simulink model "c28x_i2c_eeprom"  (R2021b)
settings: Solver=FixedStepDiscrete  StartTime=0.0  StopTime=inf  RelTol=1e-3  EnableMultiTasking=on
libraries: simulink x3, c280xlib x3, demo_controls x1, idelinklib_common x1
settings Model: SimulationMode=external  ExtModeTrigDuration=8  Creator=The MathWorks, Inc.  LastModifiedBy=The MathWorks, Inc.
settings SolverCC: AlgebraicLoopSolver=TrustRegion
settings DataIOCC: ReturnWorkspaceOutputs=off
settings OptimizationCC: DefaultUnderspecifiedDataType=single  PassReuseOutputArgsAs=Individual arguments  MaxStackSize=512  EfficientTunableParamExpr=on
settings DebuggingCC: ParameterTunabilityLossMsg=error  SFMachineParentedDataDiag=warning  ArithmeticOperatorsInVariantConditions=warning
settings HardwareCC: ProdBitPerChar=16  ProdBitPerInt=16  ProdBitPerPointer=32  ProdBitPerSizeT=32  ProdBitPerPtrDiffT=32  ProdLargestAtomicInteger=Integer  ProdLargestAtomicFloat=None  ProdWordSize=16  ProdLongLongMode=on  ProdHWDeviceType=Texas Instruments->C2000
settings SFSimCC: SimUseLocalCustomCode=off  CustomCodeUndefinedFunction=UseInterfaceOnly
settings RTWCC: Description=Embedded Coder  SystemTargetFile=ert.tlc  HardwareBoard=TI Delfino F2833x  TemplateMakefile=ert_default_tmf  GenerateReport=on  RTWUseLocalCustomCode=off  Toolchain=Texas Instruments Code Composer Studio (C2000)  IncludeHyperlinkInReport=on  LaunchReport=on  GenerateTraceInfo=on  GenerateTraceReport=on  GenerateTraceReportSl=on  GenerateTraceReportSf=on  GenerateTraceReportEml=on
settings CodeAppCC: ForceParamTrailComments=on  IgnoreCustomStorageClasses=off  OperatorAnnotations=on  SimulinkDataObjDesc=on  SFDataObjDesc=on  MATLABFcnDesc=on  InsertBlockDesc=on  StateflowObjectComments=on  MATLABSourceComments=on
settings ERTTargetCC: CodeReplacementLibrary=TI C28x  ExtModeTransport=4  ExtModeStaticAlloc=on  ExtModeStaticAllocSize=5000  ExtModeMexFile=ext_xcp  ExtModeIntrfLevel=Level2 - Open

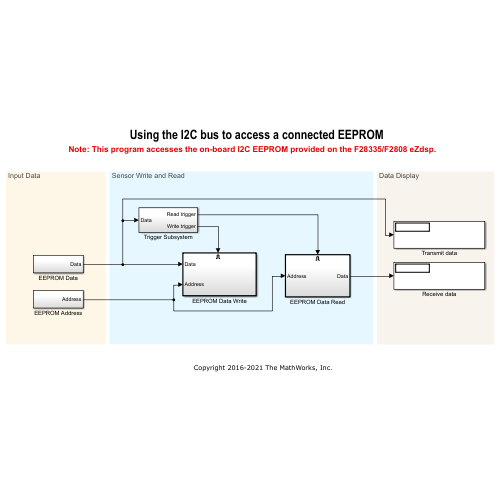
[thumbnail: Simulink's stored preview of the top-level diagram]
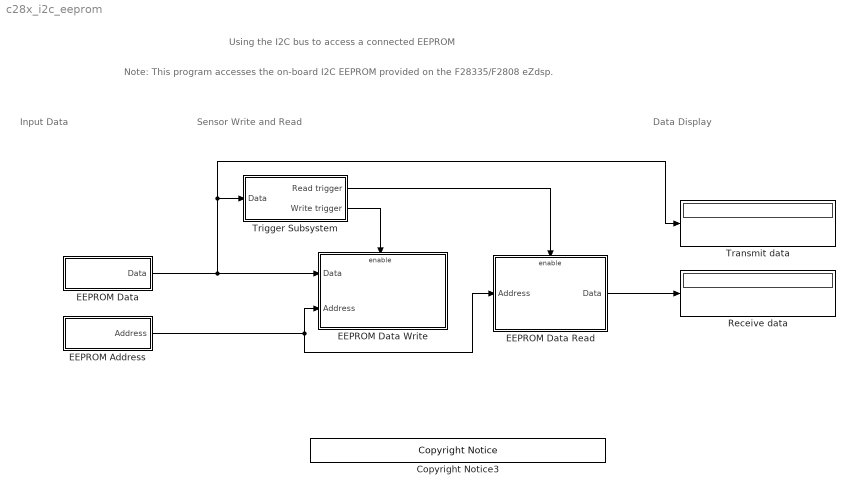
== system c28x_i2c_eeprom ==
  note: Note: This program accesses the on-board I2C EEPROM provided on the F28335/F2808 eZdsp.
  note: Using the I2C bus to access a connected EEPROM
  note: Data Display
  note: Sensor Write and Read
  note: Input Data
  Copyright Notice3 : demo_controls/Copyright Notice  year=2016  prod=tic2000
      settings: SourceProductBaseCode=ME
  EEPROM Address : Subsystem
  EEPROM Data : Subsystem
  EEPROM Data Read : Subsystem
  EEPROM Data Write : Subsystem  TreatAsAtomicUnit=on
  Receive data : Display
  Transmit data : Display
  Trigger Subsystem : Subsystem
  wires:
  EEPROM Data Read/1(Data) -> Receive data/1
  EEPROM Address/1(Address) -> EEPROM Data Read/1(Address), EEPROM Data Write/2(Address)
  EEPROM Data/1(Data) -> Transmit data/1, Trigger Subsystem/1(Data), EEPROM Data Write/1(Data)
  Trigger Subsystem/1(Read trigger) -> EEPROM Data Read/Enable
  Trigger Subsystem/2(Write trigger) -> EEPROM Data Write/Enable

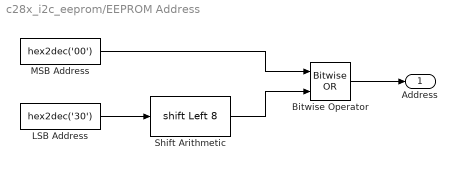
== system c28x_i2c_eeprom/EEPROM Address ==
  Bitwise Operator : simulink/Logic and Bit Operations/Bitwise Operator  logicop=OR  UseBitMask=off  NumInputPorts=2  BitMask=bin2dec('11011001')  BitMaskRealWorld=Stored Integer
  LSB Address : Constant  Value=hex2dec('30')  OutDataTypeStr=uint16  SampleTime=-1
  MSB Address : Constant  Value=hex2dec('00')  OutDataTypeStr=uint16  SampleTime=-1
  Shift Arithmetic : ArithShift  BitShiftNumber=8  BitShiftDirection=Left
  Address : Outport  VectorParamsAs1DForOutWhenUnconnected=off
  wires:
  LSB Address/1 -> Shift Arithmetic/1
  MSB Address/1 -> Bitwise Operator/1
  Shift Arithmetic/1 -> Bitwise Operator/2
  Bitwise Operator/1 -> Address/1

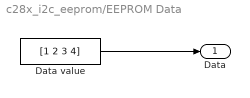
== system c28x_i2c_eeprom/EEPROM Data ==
  Data value : Constant  Value=[1 2 3 4]  OutDataTypeStr=uint16  SampleTime=-1
  Data : Outport  VectorParamsAs1DForOutWhenUnconnected=off
  wires:
  Data value/1 -> Data/1

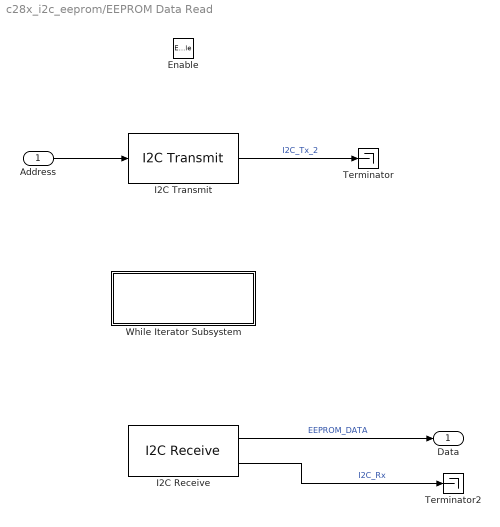
== system c28x_i2c_eeprom/EEPROM Data Read ==
  Address : Inport
  Enable : EnablePort
  I2C Receive : c280xlib/I2C Receive  Priority=3  selectModule=I2C_A  addrFormat=7-Bit addressing  saSource=Specify via dialog  SAR=hex2dec('50')  bitCount=8  dataLength=4  initValue=0  NACK=off  STP=on  STR=on  sampleTime=0.2  dataType=uint16
      settings: SourceProductBaseCode=TIC2000
  I2C Transmit : c280xlib/I2C Transmit  Priority=1  selectModule=I2C_A  addrFormat=7-Bit addressing  saSource=Specify via dialog  SAR=hex2dec('50')  bitCount=8  STP=off  RM=off  STR=on
      settings: SourceProductBaseCode=TIC2000
  Terminator : Terminator
  Terminator2 : Terminator
  While Iterator Subsystem : Subsystem  Priority=2  TreatAsAtomicUnit=on
  Data : Outport  VectorParamsAs1DForOutWhenUnconnected=off
  wires:
  I2C Receive/2 -> Terminator2/1  "I2C_Rx"
  I2C Transmit/1 -> Terminator/1  "I2C_Tx_2"
  Address/1 -> I2C Transmit/1
  I2C Receive/1 -> Data/1  "EEPROM_DATA"

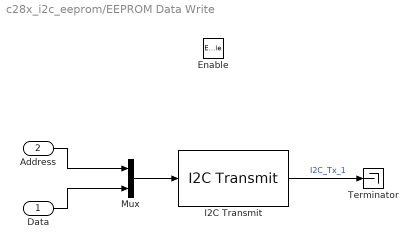
== system c28x_i2c_eeprom/EEPROM Data Write ==
  Data : Inport
  Address : Inport  Port=2
  Enable : EnablePort
  I2C Transmit : c280xlib/I2C Transmit  Priority=1  selectModule=I2C_A  addrFormat=7-Bit addressing  saSource=Specify via dialog  SAR=hex2dec('50')  bitCount=8  STP=on  RM=off  STR=on
      settings: SourceProductBaseCode=TIC2000
  Mux : Mux  Inputs=2
  Terminator : Terminator
  wires:
  I2C Transmit/1 -> Terminator/1  "I2C_Tx_1"
  Mux/1 -> I2C Transmit/1
  Data/1 -> Mux/2
  Address/1 -> Mux/1

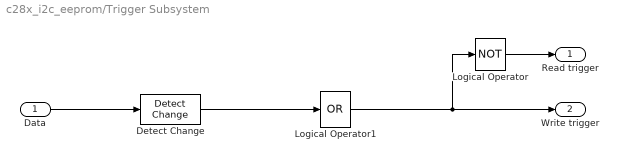
== system c28x_i2c_eeprom/Trigger Subsystem ==
  Data : Inport
  Detect Change : simulink/Logic and Bit Operations/Detect Change  vinit=0  OutDataTypeStr=boolean
  Logical Operator : Logic  Operator=NOT  AllPortsSameDT=off  OutDataTypeStr=boolean
  Logical Operator1 : Logic  Operator=OR  Inputs=1  AllPortsSameDT=off  OutDataTypeStr=boolean
  Read trigger : Outport  VectorParamsAs1DForOutWhenUnconnected=off
  Write trigger : Outport  Port=2  VectorParamsAs1DForOutWhenUnconnected=off
  wires:
  Data/1 -> Detect Change/1
  Detect Change/1 -> Logical Operator1/1
  Logical Operator1/1 -> Logical Operator/1, Write trigger/1
  Logical Operator/1 -> Read trigger/1

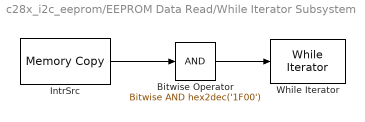
== system c28x_i2c_eeprom/EEPROM Data Read/While Iterator Subsystem ==
  Bitwise Operator : simulink/Logic and Bit Operations/Bitwise Operator  logicop=AND  UseBitMask=on  BitMask=hex2dec('1F00')  BitMaskRealWorld=Stored Integer
  IntrSrc : idelinklib_common/Memory Copy  copyFrom=Specified source code symbol  copyFromAddressSource=Specify via dialog  copyFromAddress=hex2dec('00001000')  copyFromSrcCode=&I2caRegs.I2CFFTX.all  dataTypeFrom=uint16  dataDimensionFrom=1  useOffsetFrom=off  offsetFromSrc=Specify via dialog  offsetFrom=1  strideFrom=1  copyTo=Output port  copyToAddressSource=Specify via dialog  copyToAddress=hex2dec('00002000')  copyToSrcCode=myVariableDst  dataTypeTo=uint16  useOffsetTo=off  offsetToSrc=Specify via dialog  offsetTo=1  strideTo=1  sampleTime=-1  useInitValue=off  initValueSrc=Specify constant value  initValue=1  initValueSrcCode=myInitValueVariable  useAsMask=off  maskOperator=bitwise AND  useTermValue=off  termValue=1  isRealtimeEnabled=off  emitCCBeforeWrite=off  CCBeforeWrite=/* Custom Code Before Write*/  emitCCAfterWrite=off  CCAfterWrite=/* Custom Code After Write*/  useDMACopy=off  enableBlockingMode=off
      settings: SourceProductBaseCode=ME
  While Iterator : WhileIterator  MaxIters=-1  WhileBlockType=do-while
  wires:
  IntrSrc/1 -> Bitwise Operator/1
  Bitwise Operator/1 -> While Iterator/1
